simulink model "Simulaciones"  (R2025b)
settings: Solver=VariableStepAuto  StartTime=0.0  StopTime=10.0  RelTol=1e-3
settings Model: Creator=andre  LastModifiedBy=andre

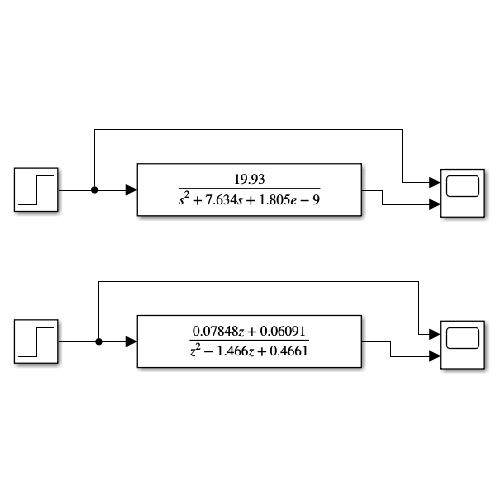
[thumbnail: Simulink's stored preview of the top-level diagram]
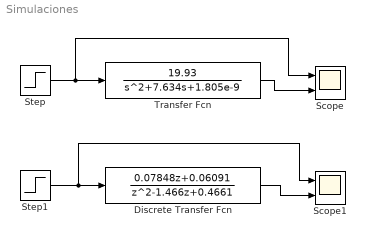
== system Simulaciones ==
  Discrete Transfer Fcn : DiscreteTransferFcn  Numerator=[0.07848 0.06091]  Denominator=[1 -1.466 0.4661]
  Scope : Scope  NumInputPorts=2
      settings: ActiveDisplayYMinimum=-0.79812355009356217  ActiveDisplayYMaximum=1.7492642479823211
  Scope1 : Scope  NumInputPorts=2
  Step : Step  Time=0  SampleTime=0
  Step1 : Step  Time=0  SampleTime=0
  Transfer Fcn : TransferFcn  Numerator=[19.93]  Denominator=[1 7.634 1.805e-9]
  wires:
  Transfer Fcn/1 -> Scope/2
  Discrete Transfer Fcn/1 -> Scope1/2
  Step/1 -> Scope/1, Transfer Fcn/1
  Step1/1 -> Discrete Transfer Fcn/1, Scope1/1
